simulink model "TTS2_EXT"  (R2025b)
settings: Solver=FixedStepAuto  StartTime=0.0  StopTime=inf  FixedStep=0.01  RelTol=1e-3
model workspace (MAT data in the model file):
  amp_f1 = -100
  amp_f10 = 0.5
  amp_f11 = -0.1
  amp_f12 = 1
  amp_f13 = 0.5
  amp_f14 = -20
  amp_f15 = 0.5
  amp_f16 = 0.5
  amp_f17 = 20
  amp_f18 = -30
  amp_f19 = 0.1
  amp_f2 = -20
  amp_f20 = -20
  amp_f21 = 20
  amp_f3 = -30
  amp_f4 = -30
  amp_f5 = -10
  amp_f51 = -10
  amp_f52 = -30
  amp_f53 = -30
  amp_f54 = 20
  amp_f55 = -100
  amp_f6 = -30
  amp_f7 = -30
  amp_f8 = -30
  amp_f9 = 1
  from_f1 = 570
  from_f10 = 5970
  from_f11 = 6570
  from_f12 = 7170
  from_f13 = 7770
  from_f14 = 8370
  from_f15 = 8970
  from_f16 = 9570
  from_f17 = 10170
  from_f18 = 10770
  from_f19 = 11370
  from_f2 = 1170
  from_f20 = 11970
  from_f21 = 12570
  from_f3 = 1770
  from_f4 = 2370
  from_f5 = 2970
  from_f51 = 13170
  from_f52 = 13770
  from_f53 = 14370
  from_f54 = 14970
  from_f55 = 15570
  from_f6 = 3570
  from_f7 = 4170
  from_f8 = 4770
  from_f9 = 5370
libraries: lab310_library x26, neural x15, simulink x4, opclib x3, fuzblock x1
(part 2 of 3)

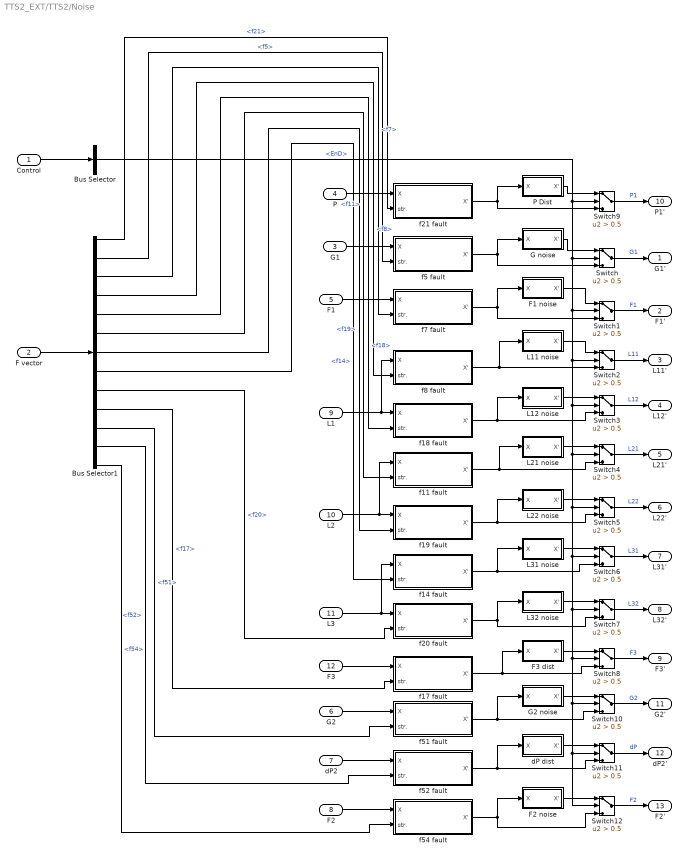
== system TTS2_EXT/TTS2/Noise ==
  Control : Inport
  F vector : Inport  Port=2
  G1 : Inport  Port=3
  P : Inport  Port=4
  F1 : Inport  Port=5
  G2 : Inport  Port=6
  dP2 : Inport  Port=7
  F2 : Inport  Port=8
  L1 : Inport  Port=9
  L2 : Inport  Port=10
  L3 : Inport  Port=11
  F3 : Inport  Port=12
  Bus Selector : BusSelector  OutputSignals=EnD
  Bus Selector1 : BusSelector  OutputSignals=f21,f5,f7,f8,f18,f11,f19,f14,f20,f17,f51,f52,f54
  F1 noise : Subsystem
  F2 noise : Subsystem
  F3 dist : Subsystem
  G noise : Subsystem
  G2 noise : Subsystem
  L11 noise : Subsystem
  L12 noise : Subsystem
  L21 noise : Subsystem
  L22 noise : Subsystem
  L31 noise : Subsystem
  L32 noise : Subsystem
  P Dist : Subsystem
  Switch{,1..12} (13 alike) : Switch  Criteria=u2 > Threshold  Threshold=0.5  SaturateOnIntegerOverflow=off  InputSameDT=off
  dP dist : Subsystem
  f11 fault : Subsystem
  f14 fault : Subsystem
  f17 fault : Subsystem
  f18 fault : Subsystem
  f19 fault : Subsystem
  f20 fault : Subsystem
  f21 fault : Subsystem
  f5 fault : Subsystem
  f51 fault : Subsystem
  f52 fault : Subsystem
  f54 fault : Subsystem
  f7 fault : Subsystem
  f8 fault : Subsystem
  G1' : Outport  VectorParamsAs1DForOutWhenUnconnected=off
  F1' : Outport  Port=2  VectorParamsAs1DForOutWhenUnconnected=off
  L11' : Outport  Port=3  VectorParamsAs1DForOutWhenUnconnected=off
  L12' : Outport  Port=4  VectorParamsAs1DForOutWhenUnconnected=off
  L21' : Outport  Port=5  VectorParamsAs1DForOutWhenUnconnected=off
  L22' : Outport  Port=6  VectorParamsAs1DForOutWhenUnconnected=off
  L31' : Outport  Port=7  VectorParamsAs1DForOutWhenUnconnected=off
  L32' : Outport  Port=8  VectorParamsAs1DForOutWhenUnconnected=off
  F3' : Outport  Port=9  VectorParamsAs1DForOutWhenUnconnected=off
  P1' : Outport  Port=10  VectorParamsAs1DForOutWhenUnconnected=off
  G2' : Outport  Port=11  VectorParamsAs1DForOutWhenUnconnected=off
  dP2' : Outport  Port=12  VectorParamsAs1DForOutWhenUnconnected=off
  F2' : Outport  Port=13  VectorParamsAs1DForOutWhenUnconnected=off
  wires:
  f21 fault/1(X') -> P Dist/1(X), Switch9/3
  P Dist/1(X') -> Switch9/1
  Switch9/1 -> P1'/1  "P1"
  P/1 -> f21 fault/1(X)
  Switch2/1 -> L11'/1  "L11"
  Switch8/1 -> F3'/1  "F3"
  Switch7/1 -> L32'/1  "L32"
  F1 noise/1(X') -> Switch1/1
  Switch3/1 -> L12'/1  "L12"
  Switch4/1 -> L21'/1  "L21"
  Switch6/1 -> L31'/1  "L31"
  L11 noise/1(X') -> Switch2/1
  G noise/1(X') -> Switch/1
  Switch5/1 -> L22'/1  "L22"
  f20 fault/1(X') -> Switch7/3, L32 noise/1(X)
  F3 dist/1(X') -> Switch8/1
  f11 fault/1(X') -> Switch4/3, L21 noise/1(X)
  L32 noise/1(X') -> Switch7/1
  L31 noise/1(X') -> Switch6/1
  f18 fault/1(X') -> Switch3/3, L12 noise/1(X)
  F1/1 -> f7 fault/1(X)
  L22 noise/1(X') -> Switch5/1
  L1/1 -> f18 fault/1(X), f8 fault/1(X)
  L2/1 -> f11 fault/1(X), f19 fault/1(X)
  Switch/1 -> G1'/1  "G1"
  f5 fault/1(X') -> Switch/3, G noise/1(X)
  L21 noise/1(X') -> Switch4/1
  f19 fault/1(X') -> Switch5/3, L22 noise/1(X)
  Bus Selector/1 -> Switch9/2, Switch8/2, Switch12/2, Switch11/2, Switch10/2, Switch7/2, Switch6/2, Switch5/2, Switch4/2, Switch3/2, Switch2/2, Switch1/2, Switch/2  "<EnD>"
  f17 fault/1(X') -> F3 dist/1(X), Switch8/3
  Switch1/1 -> F1'/1  "F1"
  L12 noise/1(X') -> Switch3/1
  f8 fault/1(X') -> Switch2/3, L11 noise/1(X)
  f14 fault/1(X') -> Switch6/3, L31 noise/1(X)
  f7 fault/1(X') -> Switch1/3, F1 noise/1(X)
  L3/1 -> f14 fault/1(X), f20 fault/1(X)
  G1/1 -> f5 fault/1(X)
  Control/1 -> Bus Selector/1
  F vector/1 -> Bus Selector1/1
  Bus Selector1/1 -> f21 fault/2(str.)  "<f21>"
  Bus Selector1/2 -> f5 fault/2(str.)  "<f5>"
  Bus Selector1/3 -> f7 fault/2(str.)  "<f7>"
  Bus Selector1/4 -> f8 fault/2(str.)  "<f8>"
  Bus Selector1/5 -> f18 fault/2(str.)  "<f18>"
  Bus Selector1/6 -> f11 fault/2(str.)  "<f11>"
  Bus Selector1/7 -> f19 fault/2(str.)  "<f19>"
  Bus Selector1/8 -> f14 fault/2(str.)  "<f14>"
  Bus Selector1/9 -> f20 fault/2(str.)  "<f20>"
  Bus Selector1/10 -> f17 fault/2(str.)  "<f17>"
  dP2/1 -> f52 fault/1(X)
  G2/1 -> f51 fault/1(X)
  Switch12/1 -> F2'/1  "F2"
  Switch11/1 -> dP2'/1  "dP"
  Switch10/1 -> G2'/1  "G2"
  f54 fault/1(X') -> F2 noise/1(X), Switch12/3
  f52 fault/1(X') -> Switch11/3, dP dist/1(X)
  f51 fault/1(X') -> Switch10/3, G2 noise/1(X)
  G2 noise/1(X') -> Switch10/1
  dP dist/1(X') -> Switch11/1
  F2 noise/1(X') -> Switch12/1
  Bus Selector1/11 -> f51 fault/2(str.)  "<f51>"
  Bus Selector1/12 -> f52 fault/2(str.)  "<f52>"
  Bus Selector1/13 -> f54 fault/2(str.)  "<f54>"
  F2/1 -> f54 fault/1(X)
  F3/1 -> f17 fault/1(X)

== system TTS2_EXT/TTS2/Pump+pipe+control valve ==
  CV1 : Inport
  F vec : Inport  Port=2
  CV2 : Inport  Port=3
  Add : Sum
  Bus Selector : BusSelector  OutputSignals=f1,f2,f4,f6,f53
  Patm[kPa] : Constant  Value=1.013  OutMin=[0.1013]  OutMax=[2.026]
  Pump control [%] : Constant  Value=pc  mask{pc=100.0}
      mask prompts: pc "Pump control"
  Pump+Pipe : Subsystem
  V1 : Subsystem
  V2 : Subsystem
  f1 fault : Subsystem
  f2 fault : Subsystem
  X1[%] : Outport  VectorParamsAs1DForOutWhenUnconnected=off
  F1[m3/s] : Outport  Port=2  VectorParamsAs1DForOutWhenUnconnected=off
  dP1[kPa] : Outport  Port=3  VectorParamsAs1DForOutWhenUnconnected=off
  P[kPa] : Outport  Port=4  VectorParamsAs1DForOutWhenUnconnected=off
  X2[%] : Outport  Port=5  VectorParamsAs1DForOutWhenUnconnected=off
  F2[m3/s] : Outport  Port=6  VectorParamsAs1DForOutWhenUnconnected=off
  dP2[kPa] : Outport  Port=7  VectorParamsAs1DForOutWhenUnconnected=off
  wires:
  Pump control [%]/1 -> f1 fault/1(X)
  f2 fault/1(Xf) -> Pump+Pipe/1(MP)
  f1 fault/1(Xf) -> f2 fault/1(X)
  Bus Selector/2 -> f2 fault/2(str.)  "<f2>"
  Bus Selector/1 -> f1 fault/2(str.)  "<f1>"
  F vec/1 -> Bus Selector/1
  Pump+Pipe/1(P[kPa]) -> P[kPa]/1, V2/2(P1[kPa]), V1/2(P1[kPa])
  CV1/1 -> V1/1(CV[%])
  Patm[kPa]/1 -> V2/3(P2[kPa]), V1/3(P2[kPa])
  Bus Selector/3 -> V1/4(f04)  "<f4>"
  Bus Selector/4 -> V1/5(f06)  "<f6>"
  V1/1(X[%]) -> X1[%]/1
  V1/3(dP[kPa]) -> dP1[kPa]/1
  V1/2(F[m3/s]) -> Add/2, F1[m3/s]/1
  CV2/1 -> V2/1(CV[%])
  V2/1(X[%]) -> X2[%]/1
  V2/2(F[m3/s]) -> Add/1, F2[m3/s]/1
  V2/3(dP[kPa]) -> dP2[kPa]/1
  Bus Selector/5 -> V2/4(f53)  "<f53>"
  Add/1 -> Pump+Pipe/2(F[m3/h])

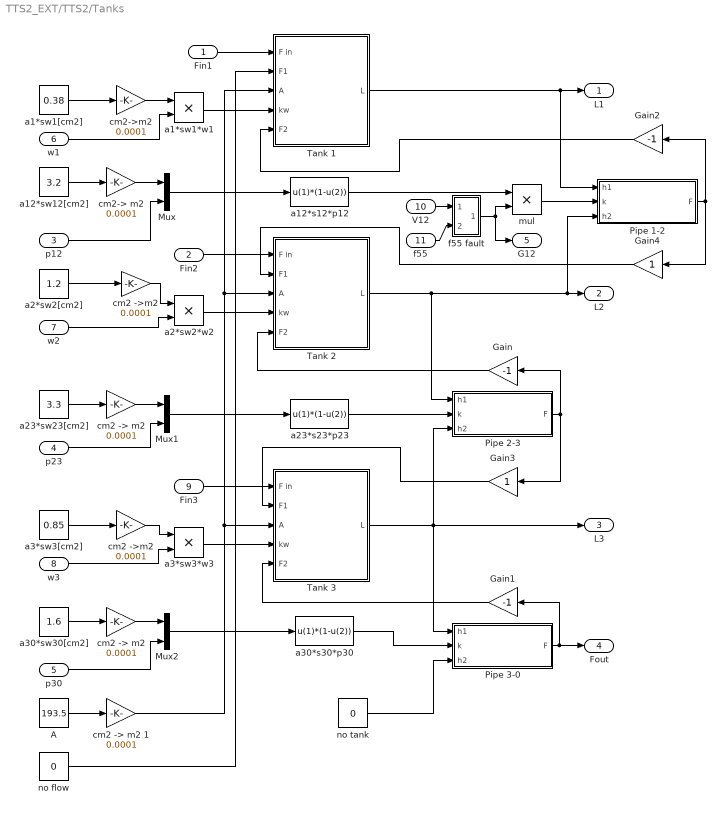
== system TTS2_EXT/TTS2/Tanks ==
  Fin1 : Inport
  Fin2 : Inport  Port=2
  p12 : Inport  Port=3
  p23 : Inport  Port=4
  p30 : Inport  Port=5
  w1 : Inport  Port=6
  w2 : Inport  Port=7
  w3 : Inport  Port=8
  Fin3 : Inport  Port=9
  V12 : Inport  Port=10
  f55 : Inport  Port=11
  A : Constant  Value=193.5
  Gain : Gain  Gain=-1
  Gain1 : Gain  Gain=-1
  Gain2 : Gain  Gain=-1
  Gain3 : Gain
  Gain4 : Gain
  Mux : Mux  Inputs=2
  Mux1 : Mux  Inputs=2
  Mux2 : Mux  Inputs=2
  Pipe 1-2 : Subsystem
  Pipe 2-3 : Subsystem
  Pipe 3-0 : Subsystem
  "Tank 1 " : Subsystem
  Tank 2 : Subsystem
  Tank 3 : Subsystem
  a1*sw1*w1 : Product
  a1*sw1[cm2] : Constant  Value=0.38
  a12*s12*p12 : Fcn  Expr=u(1)*(1-u(2))
  a12*sw12[cm2] : Constant  Value=3.2
  a2*sw2*w2 : Product
  a2*sw2[cm2] : Constant  Value=1.2
  a23*s23*p23 : Fcn  Expr=u(1)*(1-u(2))
  a23*sw23[cm2] : Constant  Value=3.3
  a3*sw3*w3 : Product
  a3*sw3[cm2] : Constant  Value=0.85
  a30*s30*p30 : Fcn  Expr=u(1)*(1-u(2))
  a30*sw30[cm2] : Constant  Value=1.6
  "cm2 -> m2" : Gain  Gain=0.0001
  "cm2 -> m2 " : Gain  Gain=0.0001
  "cm2 -> m2 1" : Gain  Gain=0.0001
  cm2 ->m2 : Gain  Gain=0.0001
  "cm2 ->m2 " : Gain  Gain=0.0001
  cm2-> m2 : Gain  Gain=0.0001
  cm2->m2 : Gain  Gain=0.0001
  f55 fault : Subsystem
  mul : Product
  no flow : Constant  Value=0
  no tank : Constant  Value=0
  L1 : Outport  VectorParamsAs1DForOutWhenUnconnected=off
  L2 : Outport  Port=2  VectorParamsAs1DForOutWhenUnconnected=off
  L3 : Outport  Port=3  VectorParamsAs1DForOutWhenUnconnected=off
  Fout : Outport  Port=4  VectorParamsAs1DForOutWhenUnconnected=off
  G12 : Outport  Port=5  VectorParamsAs1DForOutWhenUnconnected=off
  wires:
  Fin1/1 -> "Tank 1 "/1(F in)
  a1*sw1[cm2]/1 -> cm2->m2/1
  cm2->m2/1 -> a1*sw1*w1/1
  a1*sw1*w1/1 -> "Tank 1 "/4(kw)
  w1/1 -> a1*sw1*w1/2
  a12*sw12[cm2]/1 -> cm2-> m2/1
  cm2-> m2/1 -> Mux/1
  p12/1 -> Mux/2
  Mux/1 -> a12*s12*p12/1
  a2*sw2[cm2]/1 -> cm2 ->m2/1
  cm2 ->m2/1 -> a2*sw2*w2/1
  a23*sw23[cm2]/1 -> "cm2 -> m2"/1
  "cm2 -> m2"/1 -> Mux1/1
  Mux1/1 -> a23*s23*p23/1
  w2/1 -> a2*sw2*w2/2
  p23/1 -> Mux1/2
  a2*sw2*w2/1 -> Tank 2/4(kw)
  a3*sw3[cm2]/1 -> "cm2 ->m2 "/1
  "cm2 ->m2 "/1 -> a3*sw3*w3/1
  a30*sw30[cm2]/1 -> "cm2 -> m2 "/1
  "cm2 -> m2 "/1 -> Mux2/1
  w3/1 -> a3*sw3*w3/2
  p30/1 -> Mux2/2
  Mux2/1 -> a30*s30*p30/1
  a3*sw3*w3/1 -> Tank 3/4(kw)
  A/1 -> "cm2 -> m2 1"/1
  no flow/1 -> "Tank 1 "/2(F1)
  "cm2 -> m2 1"/1 -> Tank 3/3(A), Tank 2/3(A), "Tank 1 "/3(A)
  "Tank 1 "/1(L) -> Pipe 1-2/1(h1), L1/1
  a12*s12*p12/1 -> mul/1
  Tank 2/1(L) -> Pipe 1-2/3(h2), L2/1, Pipe 2-3/1(h1)
  a23*s23*p23/1 -> Pipe 2-3/2(k)
  Tank 3/1(L) -> Pipe 2-3/3(h2), Pipe 3-0/1(h1), L3/1
  a30*s30*p30/1 -> Pipe 3-0/2(k)
  no tank/1 -> Pipe 3-0/3(h2)
  Pipe 3-0/1(F) -> Fout/1, Gain1/1
  Pipe 2-3/1(F) -> Gain3/1, Gain/1
  Pipe 1-2/1(F) -> Gain2/1, Gain4/1
  Gain2/1 -> "Tank 1 "/5(F2)
  Gain/1 -> Tank 2/5(F2)
  Fin3/1 -> Tank 3/1(F in)
  Gain1/1 -> Tank 3/5(F2)
  Gain3/1 -> Tank 3/2(F1)
  Gain4/1 -> Tank 2/2(F1)
  Fin2/1 -> Tank 2/1(F in)
  mul/1 -> Pipe 1-2/2(k)
  V12/1 -> f55 fault/1(X)
  f55/1 -> f55 fault/2(str.)
  f55 fault/1(X') -> G12/1, mul/2

== system TTS2_EXT/TTS2/f3 fault ==
  X : Inport
  str. : Inport  Port=2
  Add : Sum
  Fcn : Fcn  Expr=u(1)*((u(2)/100)+1)
  Manual Switch : ManualSwitch  CurrentSetting=0
  Mux : Mux  Inputs=2
  X' : Outport  VectorParamsAs1DForOutWhenUnconnected=off
  wires:
  Mux/1 -> Fcn/1
  X/1 -> Add/1, Mux/1
  str./1 -> Add/2, Mux/2
  Manual Switch/1 -> X'/1
  Add/1 -> Manual Switch/1
  Fcn/1 -> Manual Switch/2

== system TTS2_EXT/Monitoring & Analysis/r4/Function Fitting Neural Network ==
  Input : Inport  PortDimensions=1
      mask Display: e = 0.06;c1 = [120 230 180]/255;c2 = ([120 230 180]+0)/(256+128);c3 = ([120 230 180]+128)/(256+128);patch([0 1 1 0],[0 0 1 1],c1);patch([0 1 1 1-e 1-e 0+e],[0 0 1 1-e 0+e 0+e],c2);patch([0 0 1 1-e 0+e 0+e],[0 1 1 1-e 1-e 0+e],c3);plot([0 1 1 0 0],[0 0 1 1 0]);
  Layer 1 : Subsystem
      mask Display: e = 0.06;c1 = [120 150 230]/255;c2 = ([120 150 230]+0)/383;c3 = ([120 150 230]+128)/383;patch([0 1 1 0],[0 0 1 1],c1);patch([0 1 1 1-e 1-e 0+e],[0 0 1 1-e 0+e 0+e],c2);patch([0 0 1 1-e 0+e 0+e],[0 1 1 1-e 1-e 0+e],c3);plot([0 1 1 0 0],[0 0 1 1 0]);
  Layer 2 : Subsystem
      mask Display: e = 0.06;c1 = [120 150 230]/255;c2 = ([120 150 230]+0)/383;c3 = ([120 150 230]+128)/383;patch([0 1 1 0],[0 0 1 1],c1);patch([0 1 1 1-e 1-e 0+e],[0 0 1 1-e 0+e 0+e],c2);patch([0 0 1 1-e 0+e 0+e],[0 1 1 1-e 1-e 0+e],c3);plot([0 1 1 0 0],[0 0 1 1 0]);
  Process Input 1 : Subsystem
      mask Display: e = 0.06;c1 = [120 150 230]/255;c2 = ([120 150 230]+0)/383;c3 = ([120 150 230]+128)/383;patch([0 1 1 0],[0 0 1 1],c1);patch([0 1 1 1-e 1-e 0+e],[0 0 1 1-e 0+e 0+e],c2);patch([0 0 1 1-e 0+e 0+e],[0 1 1 1-e 1-e 0+e],c3);plot([0 1 1 0 0],[0 0 1 1 0]);
  Process Output 1 : Subsystem
      mask Display: e = 0.06;c1 = [120 150 230]/255;c2 = ([120 150 230]+0)/383;c3 = ([120 150 230]+128)/383;patch([0 1 1 0],[0 0 1 1],c1);patch([0 1 1 1-e 1-e 0+e],[0 0 1 1-e 0+e 0+e],c2);patch([0 0 1 1-e 0+e 0+e],[0 1 1 1-e 1-e 0+e],c3);plot([0 1 1 0 0],[0 0 1 1 0]);
  Output : Outport  InitialOutput=0
      mask Display: e = 0.06;c1 = [120 230 180]/255;c2 = ([120 230 180]+0)/(256+128);c3 = ([120 230 180]+128)/(256+128);patch([0 1 1 0],[0 0 1 1],c1);patch([0 1 1 1-e 1-e 0+e],[0 0 1 1-e 0+e 0+e],c2);patch([0 0 1 1-e 0+e 0+e],[0 1 1 1-e 1-e 0+e],c3);plot([0 1 1 0 0],[0 0 1 1 0]);
  wires:
  Input/1 -> Process Input 1/1(x)
  Process Output 1/1(y) -> Output/1
  Process Input 1/1(p) -> Layer 1/1("p{1}")
  Layer 1/1("a{1}") -> [feedback1]
  [feedback1] -> Layer 2/1("a{1} ")
  Layer 2/1("a{2}") -> Process Output 1/1(a)

== system TTS2_EXT/Subsystem1/PID/Antiwindup ==
  CV : Inport
  Logical Operator : Logic  Operator=NOR  AllPortsSameDT=off  OutDataTypeStr=boolean
  Relational Operator : RelationalOperator  Operator=<=  OutDataTypeStr=boolean  RndMeth=Simplest  InputSameDT=off
  Relational Operator1 : RelationalOperator  OutDataTypeStr=boolean  RndMeth=Simplest  InputSameDT=off
  norm CV max : Constant
  norm CVmin : Constant  Value=0
  enable : Outport  VectorParamsAs1DForOutWhenUnconnected=off
  wires:
  norm CVmin/1 -> Relational Operator/2
  norm CV max/1 -> Relational Operator1/2
  CV/1 -> Relational Operator1/1, Relational Operator/1
  Relational Operator/1 -> Logical Operator/1
  Relational Operator1/1 -> Logical Operator/2
  Logical Operator/1 -> enable/1

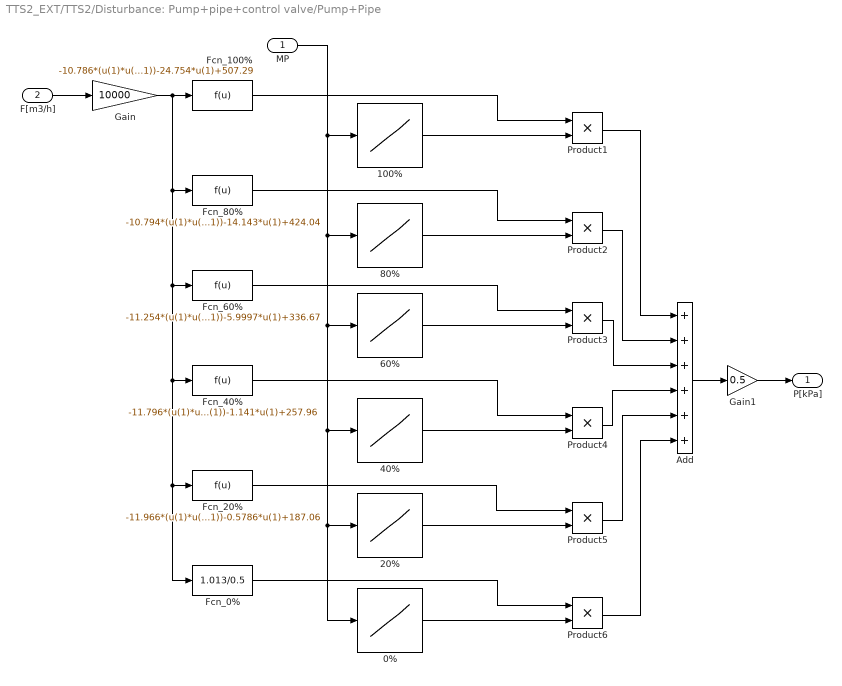
== system TTS2_EXT/TTS2/Disturbance: Pump+pipe+control valve/Pump+Pipe ==
  MP : Inport
  F[m3/h] : Inport  Port=2
  "0% " : Lookup_n-D  NumberOfTableDimensions=1  BreakpointsForDimension1=[0 20 100]  Table=[1 0 0]  InternalRulePriority=Speed  RndMeth=Simplest
  100% : Lookup_n-D  NumberOfTableDimensions=1  BreakpointsForDimension1=[0 80 100]  Table=[0 0 1]  InternalRulePriority=Speed  RndMeth=Simplest
  20% : Lookup_n-D  NumberOfTableDimensions=1  BreakpointsForDimension1=[0 20 40 100]  Table=[0 1 0 0]  InternalRulePriority=Speed  RndMeth=Simplest
  40% : Lookup_n-D  NumberOfTableDimensions=1  BreakpointsForDimension1=[0 20 40 60 100]  Table=[0 0 1 0 0]  InternalRulePriority=Speed  RndMeth=Simplest
  60% : Lookup_n-D  NumberOfTableDimensions=1  BreakpointsForDimension1=[0 40 60 80 100]  Table=[0 0 1 0 0]  InternalRulePriority=Speed  RndMeth=Simplest
  80% : Lookup_n-D  NumberOfTableDimensions=1  BreakpointsForDimension1=[0 60 80 100]  Table=[0 0 1 0]  InternalRulePriority=Speed  RndMeth=Simplest
  Add : Sum  Inputs=6
  Fcn_0% : Fcn  Expr=1.013/0.5
  Fcn_100% : Fcn  Expr=-10.786*(u(1)*u(1))-24.754*u(1)+507.29
  Fcn_20% : Fcn  Expr=-11.966*(u(1)*u(1))-0.5786*u(1)+187.06
  Fcn_40% : Fcn  Expr=-11.796*(u(1)*u(1))-1.141*u(1)+257.96
  Fcn_60% : Fcn  Expr=-11.254*(u(1)*u(1))-5.9997*u(1)+336.67
  Fcn_80% : Fcn  Expr=-10.794*(u(1)*u(1))-14.143*u(1)+424.04
  Gain : Gain  Gain=10000
  Gain1 : Gain  Gain=0.5
  Product{1..6} (6 alike) : Product
  P[kPa] : Outport  VectorParamsAs1DForOutWhenUnconnected=off
  wires:
  F[m3/h]/1 -> Gain/1
  MP/1 -> 80%/1, 40%/1, 20%/1, "0% "/1, 60%/1, 100%/1
  "0% "/1 -> Product6/2
  20%/1 -> Product5/2
  40%/1 -> Product4/2
  60%/1 -> Product3/2
  80%/1 -> Product2/2
  100%/1 -> Product1/2
  Gain/1 -> Fcn_20%/1, Fcn_0%/1, Fcn_40%/1, Fcn_60%/1, Fcn_80%/1, Fcn_100%/1
  Fcn_0%/1 -> Product6/1
  Fcn_20%/1 -> Product5/1
  Fcn_40%/1 -> Product4/1
  Fcn_60%/1 -> Product3/1
  Fcn_80%/1 -> Product2/1
  Fcn_100%/1 -> Product1/1
  Product1/1 -> Add/1
  Product2/1 -> Add/2
  Product3/1 -> Add/3
  Product4/1 -> Add/4
  Product5/1 -> Add/5
  Product6/1 -> Add/6
  Add/1 -> Gain1/1
  Gain1/1 -> P[kPa]/1

== system TTS2_EXT/TTS2/Disturbance: Pump+pipe+control valve/VB ==
  CV[%] : Inport
  P1[kPa] : Inport  Port=2
  P2[kPa] : Inport  Port=3
  Positioner : Subsystem
  Valve : Subsystem
  F[m3/h] : Outport  VectorParamsAs1DForOutWhenUnconnected=off
  wires:
  Valve/1(F[m3/h]) -> F[m3/h]/1
  P1[kPa]/1 -> Valve/2(P1[kPa])
  P2[kPa]/1 -> Valve/3(P2[kPa])
  CV[%]/1 -> Positioner/1(CV[0-100])
  Positioner/1(X[0-1]) -> Valve/1(G[0-1])

== system TTS2_EXT/TTS2/Noise/F1 noise ==
  X : Inport
  Random Number : RandomNumber  Variance=0.006889  Seed=3341  SampleTime=1
  Sum : Sum  Inputs=|++
  X' : Outport  VectorParamsAs1DForOutWhenUnconnected=off
  wires:
  Random Number/1 -> Sum/2
  X/1 -> Sum/1
  Sum/1 -> X'/1

== system TTS2_EXT/TTS2/Noise/F2 noise ==
  X : Inport
  Random Number : RandomNumber  Variance=0.0225  Seed=765756  SampleTime=1
  Sum : Sum  Inputs=|++
  X' : Outport  VectorParamsAs1DForOutWhenUnconnected=off
  wires:
  Random Number/1 -> Sum/2
  X/1 -> Sum/1
  Sum/1 -> X'/1

== system TTS2_EXT/TTS2/Noise/F3 dist ==
  X : Inport
  Random Number : RandomNumber  Variance=0.0225  Seed=756756  SampleTime=1
  Sum : Sum  Inputs=|++
  X' : Outport  VectorParamsAs1DForOutWhenUnconnected=off
  wires:
  Random Number/1 -> Sum/2
  X/1 -> Sum/1
  Sum/1 -> X'/1

== system TTS2_EXT/TTS2/Noise/G noise ==
  X : Inport
  Random Number : RandomNumber  Variance=0.006889  Seed=2312  SampleTime=1
  Sum : Sum  Inputs=|++
  X' : Outport  VectorParamsAs1DForOutWhenUnconnected=off
  wires:
  Random Number/1 -> Sum/2
  X/1 -> Sum/1
  Sum/1 -> X'/1

== system TTS2_EXT/TTS2/Noise/G2 noise ==
  X : Inport
  Random Number : RandomNumber  Variance=0.0225  Seed=75675675  SampleTime=1
  Sum : Sum  Inputs=|++
  X' : Outport  VectorParamsAs1DForOutWhenUnconnected=off
  wires:
  Random Number/1 -> Sum/2
  X/1 -> Sum/1
  Sum/1 -> X'/1

== system TTS2_EXT/TTS2/Noise/L11 noise ==
  X : Inport
  Random Number : RandomNumber  Variance=0.000002777  Seed=4324  SampleTime=1
  Sum : Sum  Inputs=|++
  X' : Outport  VectorParamsAs1DForOutWhenUnconnected=off
  wires:
  Random Number/1 -> Sum/2
  X/1 -> Sum/1
  Sum/1 -> X'/1

== system TTS2_EXT/TTS2/Noise/L12 noise ==
  X : Inport
  Random Number : RandomNumber  Variance=0.00000053777  Seed=432423  SampleTime=1
  Sum : Sum  Inputs=|++
  X' : Outport  VectorParamsAs1DForOutWhenUnconnected=off
  wires:
  Random Number/1 -> Sum/2
  X/1 -> Sum/1
  Sum/1 -> X'/1

== system TTS2_EXT/TTS2/Noise/L21 noise ==
  X : Inport
  Random Number : RandomNumber  Variance=0.000000111111111  Seed=43243423  SampleTime=1
  Sum : Sum  Inputs=|++
  X' : Outport  VectorParamsAs1DForOutWhenUnconnected=off
  wires:
  Random Number/1 -> Sum/2
  X/1 -> Sum/1
  Sum/1 -> X'/1

== system TTS2_EXT/TTS2/Noise/L22 noise ==
  X : Inport
  Random Number : RandomNumber  Variance=0.0000001111111111  Seed=32423  SampleTime=1
  Sum : Sum  Inputs=|++
  X' : Outport  VectorParamsAs1DForOutWhenUnconnected=off
  wires:
  Random Number/1 -> Sum/2
  X/1 -> Sum/1
  Sum/1 -> X'/1

== system TTS2_EXT/TTS2/Noise/L31 noise ==
  X : Inport
  Random Number : RandomNumber  Variance=0.0000017777  Seed=432454  SampleTime=1
  Sum : Sum  Inputs=|++
  X' : Outport  VectorParamsAs1DForOutWhenUnconnected=off
  wires:
  Random Number/1 -> Sum/2
  X/1 -> Sum/1
  Sum/1 -> X'/1

== system TTS2_EXT/TTS2/Noise/L32 noise ==
  X : Inport
  Random Number : RandomNumber  Variance=0.0000006944  Seed=4563565  SampleTime=1
  Sum : Sum  Inputs=|++
  X' : Outport  VectorParamsAs1DForOutWhenUnconnected=off
  wires:
  Random Number/1 -> Sum/2
  X/1 -> Sum/1
  Sum/1 -> X'/1

== system TTS2_EXT/TTS2/Noise/P Dist ==
  X : Inport
  Random Number : RandomNumber  Variance=0.09  Seed=32321  SampleTime=1
  Sum : Sum  Inputs=|++
  X' : Outport  VectorParamsAs1DForOutWhenUnconnected=off
  wires:
  Random Number/1 -> Sum/2
  X/1 -> Sum/1
  Sum/1 -> X'/1

== system TTS2_EXT/TTS2/Noise/dP dist ==
  X : Inport
  Random Number : RandomNumber  Variance=0.09  Seed=756756756  SampleTime=1
  Sum : Sum  Inputs=|++
  X' : Outport  VectorParamsAs1DForOutWhenUnconnected=off
  wires:
  Random Number/1 -> Sum/2
  X/1 -> Sum/1
  Sum/1 -> X'/1

== system TTS2_EXT/TTS2/Noise/f11 fault ==
  X : Inport
  str. : Inport  Port=2
  Add : Sum
  Fcn : Fcn  Expr=u(1)*((u(2)/100)+1)
  Manual Switch : ManualSwitch
  Mux : Mux  Inputs=2
  X' : Outport  VectorParamsAs1DForOutWhenUnconnected=off
  wires:
  Mux/1 -> Fcn/1
  X/1 -> Add/1, Mux/1
  str./1 -> Add/2, Mux/2
  Add/1 -> Manual Switch/1
  Fcn/1 -> Manual Switch/2
  Manual Switch/1 -> X'/1

== system TTS2_EXT/TTS2/Noise/f14 fault ==
  X : Inport
  str. : Inport  Port=2
  Add : Sum
  Fcn : Fcn  Expr=u(1)*((u(2)/100)+1)
  Manual Switch : ManualSwitch  CurrentSetting=0
  Mux : Mux  Inputs=2
  X' : Outport  VectorParamsAs1DForOutWhenUnconnected=off
  wires:
  Mux/1 -> Fcn/1
  X/1 -> Add/1, Mux/1
  str./1 -> Add/2, Mux/2
  Add/1 -> Manual Switch/1
  Fcn/1 -> Manual Switch/2
  Manual Switch/1 -> X'/1

== system TTS2_EXT/TTS2/Noise/f17 fault ==
  X : Inport
  str. : Inport  Port=2
  Add : Sum
  Fcn : Fcn  Expr=u(1)*((u(2)/100)+1)
  Manual Switch : ManualSwitch  CurrentSetting=0
  Mux : Mux  Inputs=2
  X' : Outport  VectorParamsAs1DForOutWhenUnconnected=off
  wires:
  Mux/1 -> Fcn/1
  X/1 -> Add/1, Mux/1
  str./1 -> Add/2, Mux/2
  Add/1 -> Manual Switch/1
  Fcn/1 -> Manual Switch/2
  Manual Switch/1 -> X'/1

== system TTS2_EXT/TTS2/Noise/f18 fault ==
  X : Inport
  str. : Inport  Port=2
  Add : Sum
  Fcn : Fcn  Expr=u(1)*((u(2)/100)+1)
  Manual Switch : ManualSwitch  CurrentSetting=0
  Mux : Mux  Inputs=2
  X' : Outport  VectorParamsAs1DForOutWhenUnconnected=off
  wires:
  Mux/1 -> Fcn/1
  X/1 -> Add/1, Mux/1
  str./1 -> Add/2, Mux/2
  Fcn/1 -> Manual Switch/2
  Manual Switch/1 -> X'/1
  Add/1 -> Manual Switch/1

== system TTS2_EXT/TTS2/Noise/f19 fault ==
  X : Inport
  str. : Inport  Port=2
  Add : Sum
  Fcn : Fcn  Expr=u(1)*((u(2)/100)+1)
  Manual Switch : ManualSwitch
  Mux : Mux  Inputs=2
  X' : Outport  VectorParamsAs1DForOutWhenUnconnected=off
  wires:
  Mux/1 -> Fcn/1
  X/1 -> Add/1, Mux/1
  str./1 -> Add/2, Mux/2
  Add/1 -> Manual Switch/1
  Fcn/1 -> Manual Switch/2
  Manual Switch/1 -> X'/1

== system TTS2_EXT/TTS2/Noise/f20 fault ==
  X : Inport
  str. : Inport  Port=2
  Add : Sum
  Fcn : Fcn  Expr=u(1)*((u(2)/100)+1)
  Manual Switch : ManualSwitch  CurrentSetting=0
  Mux : Mux  Inputs=2
  X' : Outport  VectorParamsAs1DForOutWhenUnconnected=off
  wires:
  Mux/1 -> Fcn/1
  X/1 -> Add/1, Mux/1
  str./1 -> Add/2, Mux/2
  Add/1 -> Manual Switch/1
  Fcn/1 -> Manual Switch/2
  Manual Switch/1 -> X'/1

== system TTS2_EXT/TTS2/Noise/f21 fault ==
  X : Inport
  str. : Inport  Port=2
  Add : Sum
  Fcn : Fcn  Expr=u(1)*((u(2)/100)+1)
  Manual Switch : ManualSwitch  CurrentSetting=0
  Mux : Mux  Inputs=2
  X' : Outport  VectorParamsAs1DForOutWhenUnconnected=off
  wires:
  Mux/1 -> Fcn/1
  X/1 -> Add/1, Mux/1
  str./1 -> Add/2, Mux/2
  Add/1 -> Manual Switch/1
  Fcn/1 -> Manual Switch/2
  Manual Switch/1 -> X'/1

== system TTS2_EXT/TTS2/Noise/f5 fault ==
  X : Inport
  str. : Inport  Port=2
  Add : Sum
  Fcn : Fcn  Expr=u(1)*((u(2)/100)+1)
  Manual Switch : ManualSwitch
  Mux : Mux  Inputs=2
  X' : Outport  VectorParamsAs1DForOutWhenUnconnected=off
  wires:
  Mux/1 -> Fcn/1
  X/1 -> Add/1, Mux/1
  str./1 -> Add/2, Mux/2
  Add/1 -> Manual Switch/1
  Fcn/1 -> Manual Switch/2
  Manual Switch/1 -> X'/1

== system TTS2_EXT/TTS2/Noise/f51 fault ==
  X : Inport
  str. : Inport  Port=2
  Add : Sum
  Fcn : Fcn  Expr=u(1)*((u(2)/100)+1)
  Manual Switch : ManualSwitch
  Mux : Mux  Inputs=2
  X' : Outport  VectorParamsAs1DForOutWhenUnconnected=off
  wires:
  Mux/1 -> Fcn/1
  X/1 -> Add/1, Mux/1
  str./1 -> Add/2, Mux/2
  Add/1 -> Manual Switch/1
  Fcn/1 -> Manual Switch/2
  Manual Switch/1 -> X'/1

== system TTS2_EXT/TTS2/Noise/f52 fault ==
  X : Inport
  str. : Inport  Port=2
  Add : Sum
  Fcn : Fcn  Expr=u(1)*((u(2)/100)+1)
  Manual Switch : ManualSwitch  CurrentSetting=0
  Mux : Mux  Inputs=2
  X' : Outport  VectorParamsAs1DForOutWhenUnconnected=off
  wires:
  Mux/1 -> Fcn/1
  X/1 -> Add/1, Mux/1
  str./1 -> Add/2, Mux/2
  Add/1 -> Manual Switch/1
  Fcn/1 -> Manual Switch/2
  Manual Switch/1 -> X'/1

== system TTS2_EXT/TTS2/Noise/f54 fault ==
  X : Inport
  str. : Inport  Port=2
  Add : Sum
  Fcn : Fcn  Expr=u(1)*((u(2)/100)+1)
  Manual Switch : ManualSwitch  CurrentSetting=0
  Mux : Mux  Inputs=2
  X' : Outport  VectorParamsAs1DForOutWhenUnconnected=off
  wires:
  Mux/1 -> Fcn/1
  X/1 -> Add/1, Mux/1
  str./1 -> Add/2, Mux/2
  Add/1 -> Manual Switch/1
  Fcn/1 -> Manual Switch/2
  Manual Switch/1 -> X'/1

== system TTS2_EXT/TTS2/Noise/f7 fault ==
  X : Inport
  str. : Inport  Port=2
  Add : Sum
  Fcn : Fcn  Expr=u(1)*((u(2)/100)+1)
  Manual Switch : ManualSwitch  CurrentSetting=0
  Mux : Mux  Inputs=2
  X' : Outport  VectorParamsAs1DForOutWhenUnconnected=off
  wires:
  Mux/1 -> Fcn/1
  X/1 -> Add/1, Mux/1
  str./1 -> Add/2, Mux/2
  Add/1 -> Manual Switch/1
  Fcn/1 -> Manual Switch/2
  Manual Switch/1 -> X'/1

== system TTS2_EXT/TTS2/Noise/f8 fault ==
  X : Inport
  str. : Inport  Port=2
  Add : Sum
  Fcn : Fcn  Expr=u(1)*((u(2)/100)+1)
  Manual Switch : ManualSwitch  CurrentSetting=0
  Mux : Mux  Inputs=2
  X' : Outport  VectorParamsAs1DForOutWhenUnconnected=off
  wires:
  Mux/1 -> Fcn/1
  X/1 -> Add/1, Mux/1
  str./1 -> Add/2, Mux/2
  Add/1 -> Manual Switch/1
  Fcn/1 -> Manual Switch/2
  Manual Switch/1 -> X'/1

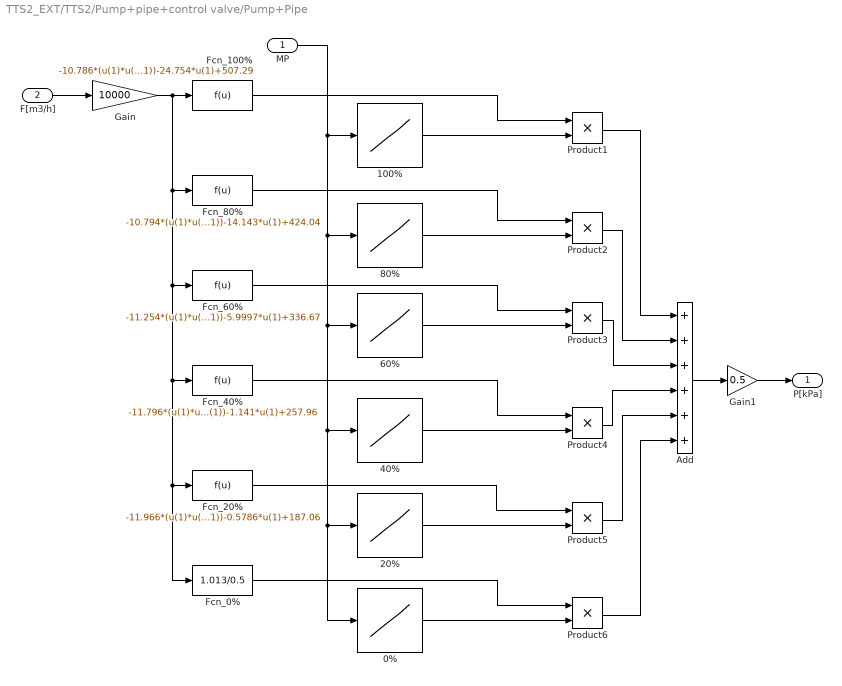
== system TTS2_EXT/TTS2/Pump+pipe+control valve/Pump+Pipe ==
  MP : Inport
  F[m3/h] : Inport  Port=2
  "0% " : Lookup_n-D  NumberOfTableDimensions=1  BreakpointsForDimension1=[0 20 100]  Table=[1 0 0]  InternalRulePriority=Speed  RndMeth=Simplest
  100% : Lookup_n-D  NumberOfTableDimensions=1  BreakpointsForDimension1=[0 80 100]  Table=[0 0 1]  InternalRulePriority=Speed  RndMeth=Simplest
  20% : Lookup_n-D  NumberOfTableDimensions=1  BreakpointsForDimension1=[0 20 40 100]  Table=[0 1 0 0]  InternalRulePriority=Speed  RndMeth=Simplest
  40% : Lookup_n-D  NumberOfTableDimensions=1  BreakpointsForDimension1=[0 20 40 60 100]  Table=[0 0 1 0 0]  InternalRulePriority=Speed  RndMeth=Simplest
  60% : Lookup_n-D  NumberOfTableDimensions=1  BreakpointsForDimension1=[0 40 60 80 100]  Table=[0 0 1 0 0]  InternalRulePriority=Speed  RndMeth=Simplest
  80% : Lookup_n-D  NumberOfTableDimensions=1  BreakpointsForDimension1=[0 60 80 100]  Table=[0 0 1 0]  InternalRulePriority=Speed  RndMeth=Simplest
  Add : Sum  Inputs=6
  Fcn_0% : Fcn  Expr=1.013/0.5
  Fcn_100% : Fcn  Expr=-10.786*(u(1)*u(1))-24.754*u(1)+507.29
  Fcn_20% : Fcn  Expr=-11.966*(u(1)*u(1))-0.5786*u(1)+187.06
  Fcn_40% : Fcn  Expr=-11.796*(u(1)*u(1))-1.141*u(1)+257.96
  Fcn_60% : Fcn  Expr=-11.254*(u(1)*u(1))-5.9997*u(1)+336.67
  Fcn_80% : Fcn  Expr=-10.794*(u(1)*u(1))-14.143*u(1)+424.04
  Gain : Gain  Gain=10000
  Gain1 : Gain  Gain=0.5
  Product{1..6} (6 alike) : Product
  P[kPa] : Outport  VectorParamsAs1DForOutWhenUnconnected=off
  wires:
  F[m3/h]/1 -> Gain/1
  MP/1 -> 80%/1, 40%/1, 20%/1, "0% "/1, 60%/1, 100%/1
  "0% "/1 -> Product6/2
  20%/1 -> Product5/2
  40%/1 -> Product4/2
  60%/1 -> Product3/2
  80%/1 -> Product2/2
  100%/1 -> Product1/2
  Gain/1 -> Fcn_20%/1, Fcn_0%/1, Fcn_40%/1, Fcn_60%/1, Fcn_80%/1, Fcn_100%/1
  Fcn_0%/1 -> Product6/1
  Fcn_20%/1 -> Product5/1
  Fcn_40%/1 -> Product4/1
  Fcn_60%/1 -> Product3/1
  Fcn_80%/1 -> Product2/1
  Fcn_100%/1 -> Product1/1
  Product1/1 -> Add/1
  Product2/1 -> Add/2
  Product3/1 -> Add/3
  Product4/1 -> Add/4
  Product5/1 -> Add/5
  Product6/1 -> Add/6
  Add/1 -> Gain1/1
  Gain1/1 -> P[kPa]/1

== system TTS2_EXT/TTS2/Pump+pipe+control valve/V1 ==
  CV[%] : Inport
  P1[kPa] : Inport  Port=2
  P2[kPa] : Inport  Port=3
  f04 : Inport  Port=4
  f06 : Inport  Port=5
  Gain2 : Gain  Gain=100
  Positioner : Subsystem
  Saturation : Saturate  UpperLimit=1  LowerLimit=0
  Valve : Subsystem
  f4 fault : Subsystem
  f6 fault : Subsystem
  X[%] : Outport  VectorParamsAs1DForOutWhenUnconnected=off
  F[m3/s] : Outport  Port=2  VectorParamsAs1DForOutWhenUnconnected=off
  dP[kPa] : Outport  Port=3  VectorParamsAs1DForOutWhenUnconnected=off
  wires:
  Valve/1(dP[kPa]) -> dP[kPa]/1
  Valve/2(F[m3/s]) -> F[m3/s]/1
  P1[kPa]/1 -> Valve/2(P1[kPa])
  P2[kPa]/1 -> Valve/3(P2[kPa])
  f06/1 -> f6 fault/2(str.)
  f6 fault/1(Xf) -> Saturation/1
  f4 fault/1(Xf) -> Positioner/1(CV[0-100])
  f04/1 -> f4 fault/2(str.)
  Positioner/1(X[0-1]) -> f6 fault/1(X), Gain2/1
  CV[%]/1 -> f4 fault/1(X)
  Gain2/1 -> X[%]/1
  Saturation/1 -> Valve/1(G[0-1])

== system TTS2_EXT/TTS2/Pump+pipe+control valve/V2 ==
  CV[%] : Inport
  P1[kPa] : Inport  Port=2
  P2[kPa] : Inport  Port=3
  f53 : Inport  Port=4
  Gain2 : Gain  Gain=100
  Positioner : Subsystem
  Saturation : Saturate  UpperLimit=1  LowerLimit=0
  Valve : Subsystem
  f53 fault : Subsystem
  X[%] : Outport  VectorParamsAs1DForOutWhenUnconnected=off
  F[m3/s] : Outport  Port=2  VectorParamsAs1DForOutWhenUnconnected=off
  dP[kPa] : Outport  Port=3  VectorParamsAs1DForOutWhenUnconnected=off
  wires:
  Valve/1(dP[kPa]) -> dP[kPa]/1
  Valve/2(F[m3/s]) -> F[m3/s]/1
  P1[kPa]/1 -> Valve/2(P1[kPa])
  P2[kPa]/1 -> Valve/3(P2[kPa])
  f53/1 -> f53 fault/2(str.)
  f53 fault/1(Xf) -> Saturation/1
  CV[%]/1 -> Positioner/1(CV[0-100])
  Positioner/1(X[0-1]) -> f53 fault/1(X), Gain2/1
  Gain2/1 -> X[%]/1
  Saturation/1 -> Valve/1(G[0-1])

== system TTS2_EXT/TTS2/Pump+pipe+control valve/f1 fault ==
  X : Inport
  str. : Inport  Port=2
  Add : Sum
  Fcn1 : Fcn  Expr=u(1)*((u(2)/100)+1)
  Manual Switch : ManualSwitch  CurrentSetting=0
  Mux1 : Mux  Inputs=2
  Xf : Outport  VectorParamsAs1DForOutWhenUnconnected=off
  wires:
  Mux1/1 -> Fcn1/1
  X/1 -> Add/1, Mux1/1
  str./1 -> Add/2, Mux1/2
  Add/1 -> Manual Switch/1
  Fcn1/1 -> Manual Switch/2
  Manual Switch/1 -> Xf/1

== system TTS2_EXT/TTS2/Pump+pipe+control valve/f2 fault ==
  X : Inport
  str. : Inport  Port=2
  Add : Sum
  Fcn : Fcn  Expr=u(1)*((u(2)/100)+1)
  Manual Switch : ManualSwitch  CurrentSetting=0
  Mux : Mux  Inputs=2
  Xf : Outport  VectorParamsAs1DForOutWhenUnconnected=off
  wires:
  Mux/1 -> Fcn/1
  X/1 -> Add/1, Mux/1
  str./1 -> Add/2, Mux/2
  Add/1 -> Manual Switch/1
  Fcn/1 -> Manual Switch/2
  Manual Switch/1 -> Xf/1

== system TTS2_EXT/TTS2/Tanks/Pipe 1-2 ==
  h1 : Inport
  k : Inport  Port=2
  h2 : Inport  Port=3
  Fcn : Fcn  Expr=sqrt(abs(u(1)*2*9.81))
  Product : Product  Inputs=3
  Sign : Signum
  Subtract : Sum  Inputs=+-
  F : Outport  VectorParamsAs1DForOutWhenUnconnected=off
  wires:
  h1/1 -> Subtract/1
  h2/1 -> Subtract/2
  Subtract/1 -> Sign/1, Fcn/1
  Fcn/1 -> Product/1
  Sign/1 -> Product/2
  k/1 -> Product/3
  Product/1 -> F/1

== system TTS2_EXT/TTS2/Tanks/Pipe 2-3 ==
  h1 : Inport
  k : Inport  Port=2
  h2 : Inport  Port=3
  Fcn : Fcn  Expr=sqrt(abs(u(1)*2*9.81))
  Product : Product  Inputs=3
  Sign : Signum
  Subtract : Sum  Inputs=+-
  F : Outport  VectorParamsAs1DForOutWhenUnconnected=off
  wires:
  h1/1 -> Subtract/1
  h2/1 -> Subtract/2
  Subtract/1 -> Sign/1, Fcn/1
  Fcn/1 -> Product/1
  Sign/1 -> Product/2
  k/1 -> Product/3
  Product/1 -> F/1

== system TTS2_EXT/TTS2/Tanks/Pipe 3-0 ==
  h1 : Inport
  k : Inport  Port=2
  h2 : Inport  Port=3
  Fcn : Fcn  Expr=sqrt(abs(u(1)*2*9.81))
  Product : Product  Inputs=3
  Sign : Signum
  Subtract : Sum  Inputs=+-
  F : Outport  VectorParamsAs1DForOutWhenUnconnected=off
  wires:
  h1/1 -> Subtract/1
  h2/1 -> Subtract/2
  Subtract/1 -> Sign/1, Fcn/1
  Fcn/1 -> Product/1
  Sign/1 -> Product/2
  k/1 -> Product/3
  Product/1 -> F/1

== system TTS2_EXT/TTS2/Tanks/Tank 1  ==
  F in : Inport
  F1 : Inport  Port=2
  A : Inport  Port=3
  kw : Inport  Port=4
  F2 : Inport  Port=5
  Divide : Product  Inputs=*/
  Gain : Gain  Gain=19.62
  Integrator : Integrator  LimitOutput=on  UpperSaturationLimit=1  LowerSaturationLimit=0
  Sqrt : Sqrt
  Subtract : Sum  Inputs=+++-
  multiply : Product  Inputs=**
  L : Outport  VectorParamsAs1DForOutWhenUnconnected=off
  wires:
  F in/1 -> Subtract/1
  F1/1 -> Subtract/2
  F2/1 -> Subtract/3
  Subtract/1 -> Divide/1
  A/1 -> Divide/2
  Divide/1 -> Integrator/1
  Integrator/1 -> Gain/1, L/1
  kw/1 -> multiply/1
  Sqrt/1 -> multiply/2
  Gain/1 -> Sqrt/1
  multiply/1 -> Subtract/4

== system TTS2_EXT/TTS2/Tanks/Tank 2 ==
  F in : Inport
  F1 : Inport  Port=2
  A : Inport  Port=3
  kw : Inport  Port=4
  F2 : Inport  Port=5
  Divide : Product  Inputs=*/
  Gain : Gain  Gain=19.62
  Integrator : Integrator  LimitOutput=on  UpperSaturationLimit=1  LowerSaturationLimit=0
  Sqrt : Sqrt
  Subtract : Sum  Inputs=+++-
  multiply : Product  Inputs=**
  L : Outport  VectorParamsAs1DForOutWhenUnconnected=off
  wires:
  F in/1 -> Subtract/1
  F1/1 -> Subtract/2
  F2/1 -> Subtract/3
  Subtract/1 -> Divide/1
  A/1 -> Divide/2
  Divide/1 -> Integrator/1
  Integrator/1 -> Gain/1, L/1
  kw/1 -> multiply/1
  Sqrt/1 -> multiply/2
  Gain/1 -> Sqrt/1
  multiply/1 -> Subtract/4

== system TTS2_EXT/TTS2/Tanks/Tank 3 ==
  F in : Inport
  F1 : Inport  Port=2
  A : Inport  Port=3
  kw : Inport  Port=4
  F2 : Inport  Port=5
  Divide : Product  Inputs=*/
  Gain : Gain  Gain=19.62
  Integrator : Integrator  LimitOutput=on  UpperSaturationLimit=1  LowerSaturationLimit=0
  Sqrt : Sqrt
  Subtract : Sum  Inputs=+++-
  multiply : Product  Inputs=**
  L : Outport  VectorParamsAs1DForOutWhenUnconnected=off
  wires:
  F in/1 -> Subtract/1
  F1/1 -> Subtract/2
  F2/1 -> Subtract/3
  Subtract/1 -> Divide/1
  A/1 -> Divide/2
  Divide/1 -> Integrator/1
  Integrator/1 -> Gain/1, L/1
  kw/1 -> multiply/1
  Sqrt/1 -> multiply/2
  Gain/1 -> Sqrt/1
  multiply/1 -> Subtract/4

== system TTS2_EXT/TTS2/Tanks/f55 fault ==
  X : Inport
  str. : Inport  Port=2
  Logical Operator : Logic  Operator=NOT  AllPortsSameDT=off  OutDataTypeStr=boolean
  Switch2 : Switch  Criteria=u2 > Threshold  SaturateOnIntegerOverflow=off  InputSameDT=off
  X' : Outport  VectorParamsAs1DForOutWhenUnconnected=off
  wires:
  Switch2/1 -> X'/1
  str./1 -> Switch2/2
  X/1 -> Switch2/3, Logical Operator/1
  Logical Operator/1 -> Switch2/1

== system TTS2_EXT/Monitoring & Analysis/r4/Function Fitting Neural Network/Layer 1 ==
  "p{1}" : Inport  PortDimensions=1
      mask Display: e = 0.06;c1 = [120 230 180]/255;c2 = ([120 230 180]+0)/(256+128);c3 = ([120 230 180]+128)/(256+128);patch([0 1 1 0],[0 0 1 1],c1);patch([0 1 1 1-e 1-e 0+e],[0 0 1 1-e 0+e 0+e],c2);patch([0 0 1 1-e 0+e 0+e],[0 1 1 1-e 1-e 0+e],c3);plot([0 1 1 0 0],[0 0 1 1 0]);
  Delays 1 : Subsystem
      mask Display: e = 0.06;c1 = [120 150 230]/255;c2 = ([120 150 230]+0)/383;c3 = ([120 150 230]+128)/383;patch([0 1 1 0],[0 0 1 1],c1);patch([0 1 1 1-e 1-e 0+e],[0 0 1 1-e 0+e 0+e],c2);patch([0 0 1 1-e 0+e 0+e],[0 1 1 1-e 1-e 0+e],c3);plot([0 1 1 0 0],[0 0 1 1 0]);disp('0');
  "IW{1,1}" : Subsystem
      mask Display: e = 0.06;c1 = [120 150 230]/255;c2 = ([120 150 230]+0)/383;c3 = ([120 150 230]+128)/383;patch([0 1 1 0],[0 0 1 1],c1);patch([0 1 1 1-e 1-e 0+e],[0 0 1 1-e 0+e 0+e],c2);patch([0 0 1 1-e 0+e 0+e],[0 1 1 1-e 1-e 0+e],c3);plot([0 1 1 0 0],[0 0 1 1 0]);disp('W');
  "b{1}" : Constant  Value=[12.5595032628997866908093783422373235225677490234375;9.0137408913545211675000246032141149044036865234375;-5.99437740726605117203007466741837561130523681640625;-4.31427156863327265767793505801819264888763427734375;0.23078101359262970238006573708844371140003204345703125;-1.3307554044509910529114904420566745102405548095703125;-3.269583881676725756193491179146803915500640869140625;-4.22281736818375730280195057275705039501190185546875;-10.9485419073701226722050705575384199619293212890625;17.15112561779046274068605271168053150177001953125]
      mask Display: e = 0.06;c1 = [120 150 230]/255;c2 = ([120 150 230]+0)/383;c3 = ([120 150 230]+128)/383;patch([0 1 1 0],[0 0 1 1],c1);patch([0 1 1 1-e 1-e 0+e],[0 0 1 1-e 0+e 0+e],c2);patch([0 0 1 1-e 0+e 0+e],[0 1 1 1-e 1-e 0+e],c3);plot([0 1 1 0 0],[0 0 1 1 0]);disp('b');
  netsum : Sum  Inputs=2  InputSameDT=on  SaturateOnIntegerOverflow=on  OutDataTypeStr=Inherit: Same as first input
      mask Display: e = 0.06;c1 = [120 150 230]/255;c2 = ([120 150 230]+0)/383;c3 = ([120 150 230]+128)/383;patch([0 1 1 0],[0 0 1 1],c1);patch([0 1 1 1-e 1-e 0+e],[0 0 1 1-e 0+e 0+e],c2);patch([0 0 1 1-e 0+e 0+e],[0 1 1 1-e 1-e 0+e],c3);plot([0 1 1 0 0],[0 0 1 1 0]);disp('+');
  tansig : neural/Transfer Functions/tansig
  "a{1}" : Outport  InitialOutput=[0;0;0;0;0;0;0;0;0;0]
      mask Display: e = 0.06;c1 = [120 230 180]/255;c2 = ([120 230 180]+0)/(256+128);c3 = ([120 230 180]+128)/(256+128);patch([0 1 1 0],[0 0 1 1],c1);patch([0 1 1 1-e 1-e 0+e],[0 0 1 1-e 0+e 0+e],c2);patch([0 0 1 1-e 0+e 0+e],[0 1 1 1-e 1-e 0+e],c3);plot([0 1 1 0 0],[0 0 1 1 0]);
  wires:
  "p{1}"/1 -> Delays 1/1("p{1}")
  Delays 1/1("pd{1,1}") -> "IW{1,1}"/1("pd{1,1}")
  "IW{1,1}"/1("iz{1,1}") -> netsum/1
  "b{1}"/1 -> netsum/2
  netsum/1 -> tansig/1
  tansig/1 -> "a{1}"/1

== system TTS2_EXT/Monitoring & Analysis/r4/Function Fitting Neural Network/Layer 2 ==
  "a{1} " : Inport  PortDimensions=10
      mask Display: e = 0.06;c1 = [120 230 180]/255;c2 = ([120 230 180]+0)/(256+128);c3 = ([120 230 180]+128)/(256+128);patch([0 1 1 0],[0 0 1 1],c1);patch([0 1 1 1-e 1-e 0+e],[0 0 1 1-e 0+e 0+e],c2);patch([0 0 1 1-e 0+e 0+e],[0 1 1 1-e 1-e 0+e],c3);plot([0 1 1 0 0],[0 0 1 1 0]);
  Delays 1 : Subsystem
      mask Display: e = 0.06;c1 = [120 150 230]/255;c2 = ([120 150 230]+0)/383;c3 = ([120 150 230]+128)/383;patch([0 1 1 0],[0 0 1 1],c1);patch([0 1 1 1-e 1-e 0+e],[0 0 1 1-e 0+e 0+e],c2);patch([0 0 1 1-e 0+e 0+e],[0 1 1 1-e 1-e 0+e],c3);plot([0 1 1 0 0],[0 0 1 1 0]);disp('0');
  "LW{2,1}" : Subsystem
      mask Display: e = 0.06;c1 = [120 150 230]/255;c2 = ([120 150 230]+0)/383;c3 = ([120 150 230]+128)/383;patch([0 1 1 0],[0 0 1 1],c1);patch([0 1 1 1-e 1-e 0+e],[0 0 1 1-e 0+e 0+e],c2);patch([0 0 1 1-e 0+e 0+e],[0 1 1 1-e 1-e 0+e],c3);plot([0 1 1 0 0],[0 0 1 1 0]);disp('W');
  "b{2}" : Constant  Value=-1.476985233725619739431067500845529139041900634765625
      mask Display: e = 0.06;c1 = [120 150 230]/255;c2 = ([120 150 230]+0)/383;c3 = ([120 150 230]+128)/383;patch([0 1 1 0],[0 0 1 1],c1);patch([0 1 1 1-e 1-e 0+e],[0 0 1 1-e 0+e 0+e],c2);patch([0 0 1 1-e 0+e 0+e],[0 1 1 1-e 1-e 0+e],c3);plot([0 1 1 0 0],[0 0 1 1 0]);disp('b');
  netsum : Sum  Inputs=2  InputSameDT=on  SaturateOnIntegerOverflow=on  OutDataTypeStr=Inherit: Same as first input
      mask Display: e = 0.06;c1 = [120 150 230]/255;c2 = ([120 150 230]+0)/383;c3 = ([120 150 230]+128)/383;patch([0 1 1 0],[0 0 1 1],c1);patch([0 1 1 1-e 1-e 0+e],[0 0 1 1-e 0+e 0+e],c2);patch([0 0 1 1-e 0+e 0+e],[0 1 1 1-e 1-e 0+e],c3);plot([0 1 1 0 0],[0 0 1 1 0]);disp('+');
  purelin : neural/Transfer Functions/purelin
  "a{2}" : Outport  InitialOutput=0
      mask Display: e = 0.06;c1 = [120 230 180]/255;c2 = ([120 230 180]+0)/(256+128);c3 = ([120 230 180]+128)/(256+128);patch([0 1 1 0],[0 0 1 1],c1);patch([0 1 1 1-e 1-e 0+e],[0 0 1 1-e 0+e 0+e],c2);patch([0 0 1 1-e 0+e 0+e],[0 1 1 1-e 1-e 0+e],c3);plot([0 1 1 0 0],[0 0 1 1 0]);
  wires:
  "a{1} "/1 -> Delays 1/1("p{2}")
  Delays 1/1("pd{2,1}") -> "LW{2,1}"/1("ad{2,1}")
  "LW{2,1}"/1("lz{2,1}") -> netsum/1
  "b{2}"/1 -> netsum/2
  netsum/1 -> purelin/1
  purelin/1 -> "a{2}"/1

== system TTS2_EXT/Monitoring & Analysis/r4/Function Fitting Neural Network/Process Input 1 ==
  x : Inport  PortDimensions=1
      mask Display: e = 0.06;c1 = [120 230 180]/255;c2 = ([120 230 180]+0)/(256+128);c3 = ([120 230 180]+128)/(256+128);patch([0 1 1 0],[0 0 1 1],c1);patch([0 1 1 1-e 1-e 0+e],[0 0 1 1-e 0+e 0+e],c2);patch([0 0 1 1-e 0+e 0+e],[0 1 1 1-e 1-e 0+e],c3);plot([0 1 1 0 0],[0 0 1 1 0]);
  mapminmax : neural/Processing Functions/mapminmax  xmin=-0.000236846370144925318784734358246  xmax=0.396988688383906829226788204323  ymin=-1  ymax=1
  p : Outport  PortDimensions=1
      mask Display: e = 0.06;c1 = [120 230 180]/255;c2 = ([120 230 180]+0)/(256+128);c3 = ([120 230 180]+128)/(256+128);patch([0 1 1 0],[0 0 1 1],c1);patch([0 1 1 1-e 1-e 0+e],[0 0 1 1-e 0+e 0+e],c2);patch([0 0 1 1-e 0+e 0+e],[0 1 1 1-e 1-e 0+e],c3);plot([0 1 1 0 0],[0 0 1 1 0]);
  wires:
  x/1 -> mapminmax/1
  mapminmax/1 -> p/1

== system TTS2_EXT/Monitoring & Analysis/r4/Function Fitting Neural Network/Process Output 1 ==
  a : Inport  PortDimensions=1
      mask Display: e = 0.06;c1 = [120 230 180]/255;c2 = ([120 230 180]+0)/(256+128);c3 = ([120 230 180]+128)/(256+128);patch([0 1 1 0],[0 0 1 1],c1);patch([0 1 1 1-e 1-e 0+e],[0 0 1 1-e 0+e 0+e],c2);patch([0 0 1 1-e 0+e 0+e],[0 1 1 1-e 1-e 0+e],c3);plot([0 1 1 0 0],[0 0 1 1 0]);
  mapminmax_reverse : neural/Processing Functions/mapminmax_reverse  xmin=-0.193966527130200377948554546492  xmax=27.2201044919786632192426623078  ymin=-1  ymax=1
  y : Outport  PortDimensions=1
      mask Display: e = 0.06;c1 = [120 230 180]/255;c2 = ([120 230 180]+0)/(256+128);c3 = ([120 230 180]+128)/(256+128);patch([0 1 1 0],[0 0 1 1],c1);patch([0 1 1 1-e 1-e 0+e],[0 0 1 1-e 0+e 0+e],c2);patch([0 0 1 1-e 0+e 0+e],[0 1 1 1-e 1-e 0+e],c3);plot([0 1 1 0 0],[0 0 1 1 0]);
  wires:
  a/1 -> mapminmax_reverse/1
  mapminmax_reverse/1 -> y/1

== system TTS2_EXT/TTS2/Disturbance: Pump+pipe+control valve/VB/Positioner ==
  CV[0-100] : Inport
  Gain : Gain  Gain=0.01
  inertia : TransferFcn  Denominator=[0.1 1]
  X[0-1] : Outport  VectorParamsAs1DForOutWhenUnconnected=off
  wires:
  CV[0-100]/1 -> Gain/1
  Gain/1 -> inertia/1
  inertia/1 -> X[0-1]/1

== system TTS2_EXT/TTS2/Disturbance: Pump+pipe+control valve/VB/Valve ==
  G[0-1] : Inport
  P1[kPa] : Inport  Port=2
  P2[kPa] : Inport  Port=3
  Abs : Abs  SaturateOnIntegerOverflow=off
  Bus Creator : BusCreator  Inputs=4
  Product : Product
  Saturation : Saturate  UpperLimit=1  LowerLimit=0
  Sign : Signum
  Sum : Sum  Inputs=|+-
  Sum1 : Sum  Inputs=|+-
  Switch : Switch  Criteria=u2 > Threshold  SaturateOnIntegerOverflow=off  InputSameDT=off
  Transfer Fcn : TransferFcn  Denominator=[1 1]
  alfa : Constant
  kv_max : Constant  Value=0.000075
  lin_range : Constant
  liniowa : Subsystem
  ro : Constant
  stałoproc. : Subsystem
  F[m3/h] : Outport  VectorParamsAs1DForOutWhenUnconnected=off
  wires:
  G[0-1]/1 -> Saturation/1
  Saturation/1 -> liniowa/1(CV), stałoproc./1(CV), Sum/1
  P1[kPa]/1 -> Sum1/1
  P2[kPa]/1 -> Sum1/2
  Sum1/1 -> Sign/1, Abs/1
  kv_max/1 -> Bus Creator/1
  alfa/1 -> Bus Creator/2
  lin_range/1 -> Bus Creator/4, Sum/2
  ro/1 -> Bus Creator/3
  Switch/1 -> Product/1
  Product/1 -> Transfer Fcn/1
  Transfer Fcn/1 -> F[m3/h]/1
  Bus Creator/1 -> liniowa/3(param), stałoproc./3(param)
  Abs/1 -> liniowa/2(dP), stałoproc./2(dP)
  Sum/1 -> Switch/2
  Sign/1 -> Product/2
  stałoproc./1(F) -> Switch/1
  liniowa/1(F) -> Switch/3

== system TTS2_EXT/TTS2/Pump+pipe+control valve/V1/Positioner ==
  CV[0-100] : Inport
  Gain : Gain  Gain=0.01
  Saturation : Saturate  UpperLimit=1  LowerLimit=0
  inertia : TransferFcn  Denominator=[0.1 1]
  X[0-1] : Outport  VectorParamsAs1DForOutWhenUnconnected=off
  wires:
  CV[0-100]/1 -> Gain/1
  Gain/1 -> inertia/1
  inertia/1 -> Saturation/1
  Saturation/1 -> X[0-1]/1

== system TTS2_EXT/TTS2/Pump+pipe+control valve/V1/Valve ==
  G[0-1] : Inport
  P1[kPa] : Inport  Port=2
  P2[kPa] : Inport  Port=3
  Abs : Abs  SaturateOnIntegerOverflow=off
  Bus Creator : BusCreator  Inputs=4
  Product : Product
  Saturation : Saturate  UpperLimit=1  LowerLimit=0
  Sign : Signum
  Sum : Sum  Inputs=|+-
  Sum1 : Sum  Inputs=|+-
  Switch : Switch  Criteria=u2 > Threshold  SaturateOnIntegerOverflow=off  InputSameDT=off
  Transfer Fcn : TransferFcn  Denominator=[1 1]
  alfa : Constant  Value=2
  kv_max : Constant  Value=0.00049
  lin_range : Constant  Value=0.1
  liniowa : Subsystem
  ro : Constant
  stałoproc. : Subsystem
  dP[kPa] : Outport  VectorParamsAs1DForOutWhenUnconnected=off
  F[m3/s] : Outport  Port=2  VectorParamsAs1DForOutWhenUnconnected=off
  wires:
  G[0-1]/1 -> Saturation/1
  Saturation/1 -> liniowa/1(CV), stałoproc./1(CV), Sum/1
  P1[kPa]/1 -> Sum1/1
  P2[kPa]/1 -> Sum1/2
  Sum1/1 -> dP[kPa]/1, Sign/1, Abs/1
  kv_max/1 -> Bus Creator/1
  alfa/1 -> Bus Creator/2
  lin_range/1 -> Bus Creator/4, Sum/2
  ro/1 -> Bus Creator/3
  Switch/1 -> Product/1
  Product/1 -> Transfer Fcn/1
  Transfer Fcn/1 -> F[m3/s]/1
  Bus Creator/1 -> liniowa/3(param), stałoproc./3(param)
  Abs/1 -> liniowa/2(dP), stałoproc./2(dP)
  Sum/1 -> Switch/2
  Sign/1 -> Product/2
  stałoproc./1(F) -> Switch/1
  liniowa/1(F) -> Switch/3

== system TTS2_EXT/TTS2/Pump+pipe+control valve/V1/f4 fault ==
  X : Inport
  str. : Inport  Port=2
  Add : Sum
  Fcn : Fcn  Expr=u(1)*((u(2)/100)+1)
  Manual Switch : ManualSwitch  CurrentSetting=0
  Mux : Mux  Inputs=2
  Xf : Outport  VectorParamsAs1DForOutWhenUnconnected=off
  wires:
  Mux/1 -> Fcn/1
  X/1 -> Add/1, Mux/1
  str./1 -> Add/2, Mux/2
  Add/1 -> Manual Switch/1
  Fcn/1 -> Manual Switch/2
  Manual Switch/1 -> Xf/1

== system TTS2_EXT/TTS2/Pump+pipe+control valve/V1/f6 fault ==
  X : Inport
  str. : Inport  Port=2
  Add : Sum
  Fcn : Fcn  Expr=u(1)*((u(2)/100)+1)
  Manual Switch : ManualSwitch  CurrentSetting=0
  Mux : Mux  Inputs=2
  Xf : Outport  VectorParamsAs1DForOutWhenUnconnected=off
  wires:
  Mux/1 -> Fcn/1
  X/1 -> Add/1, Mux/1
  str./1 -> Add/2, Mux/2
  Add/1 -> Manual Switch/1
  Fcn/1 -> Manual Switch/2
  Manual Switch/1 -> Xf/1

== system TTS2_EXT/TTS2/Pump+pipe+control valve/V2/Positioner ==
  CV[0-100] : Inport
  Gain : Gain  Gain=0.01
  Saturation : Saturate  UpperLimit=1  LowerLimit=0
  inertia : TransferFcn  Denominator=[0.1 1]
  X[0-1] : Outport  VectorParamsAs1DForOutWhenUnconnected=off
  wires:
  CV[0-100]/1 -> Gain/1
  Gain/1 -> inertia/1
  inertia/1 -> Saturation/1
  Saturation/1 -> X[0-1]/1

== system TTS2_EXT/TTS2/Pump+pipe+control valve/V2/Valve ==
  G[0-1] : Inport
  P1[kPa] : Inport  Port=2
  P2[kPa] : Inport  Port=3
  Abs : Abs  SaturateOnIntegerOverflow=off
  Bus Creator : BusCreator  Inputs=4
  Product : Product
  Saturation : Saturate  UpperLimit=1  LowerLimit=0
  Sign : Signum
  Sum : Sum  Inputs=|+-
  Sum1 : Sum  Inputs=|+-
  Switch : Switch  Criteria=u2 > Threshold  SaturateOnIntegerOverflow=off  InputSameDT=off
  Transfer Fcn : TransferFcn  Denominator=[1 1]
  alfa : Constant  Value=2
  kv_max : Constant  Value=0.00049
  lin_range : Constant  Value=0.1
  liniowa : Subsystem
  ro : Constant
  stałoproc. : Subsystem
  dP[kPa] : Outport  VectorParamsAs1DForOutWhenUnconnected=off
  F[m3/s] : Outport  Port=2  VectorParamsAs1DForOutWhenUnconnected=off
  wires:
  G[0-1]/1 -> Saturation/1
  Saturation/1 -> liniowa/1(CV), stałoproc./1(CV), Sum/1
  P1[kPa]/1 -> Sum1/1
  P2[kPa]/1 -> Sum1/2
  Sum1/1 -> dP[kPa]/1, Sign/1, Abs/1
  kv_max/1 -> Bus Creator/1
  alfa/1 -> Bus Creator/2
  lin_range/1 -> Bus Creator/4, Sum/2
  ro/1 -> Bus Creator/3
  Switch/1 -> Product/1
  Product/1 -> Transfer Fcn/1
  Transfer Fcn/1 -> F[m3/s]/1
  Bus Creator/1 -> liniowa/3(param), stałoproc./3(param)
  Abs/1 -> liniowa/2(dP), stałoproc./2(dP)
  Sum/1 -> Switch/2
  Sign/1 -> Product/2
  stałoproc./1(F) -> Switch/1
  liniowa/1(F) -> Switch/3

== system TTS2_EXT/TTS2/Pump+pipe+control valve/V2/f53 fault ==
  X : Inport
  str. : Inport  Port=2
  Add : Sum
  Fcn : Fcn  Expr=u(1)*((u(2)/100)+1)
  Manual Switch : ManualSwitch
  Mux : Mux  Inputs=2
  Xf : Outport  VectorParamsAs1DForOutWhenUnconnected=off
  wires:
  Mux/1 -> Fcn/1
  X/1 -> Add/1, Mux/1
  str./1 -> Add/2, Mux/2
  Add/1 -> Manual Switch/1
  Fcn/1 -> Manual Switch/2
  Manual Switch/1 -> Xf/1

== system TTS2_EXT/Monitoring & Analysis/r4/Function Fitting Neural Network/Layer 1/Delays 1 ==
  "p{1}" : Inport  PortDimensions=1
      mask Display: e = 0.06;c1 = [120 230 180]/255;c2 = ([120 230 180]+0)/(256+128);c3 = ([120 230 180]+128)/(256+128);patch([0 1 1 0],[0 0 1 1],c1);patch([0 1 1 1-e 1-e 0+e],[0 0 1 1-e 0+e 0+e],c2);patch([0 0 1 1-e 0+e 0+e],[0 1 1 1-e 1-e 0+e],c3);plot([0 1 1 0 0],[0 0 1 1 0]);
  mux : Mux  Inputs=1
      mask Display: e = 0.06;c1 = [120 150 230]/255;c2 = ([120 150 230]+0)/383;c3 = ([120 150 230]+128)/383;patch([0 1 1 0],[0 0 1 1],c1);patch([0 1 1 1-e 1-e 0+e],[0 0 1 1-e 0+e 0+e],c2);patch([0 0 1 1-e 0+e 0+e],[0 1 1 1-e 1-e 0+e],c3);plot([0 1 1 0 0],[0 0 1 1 0]);disp('Mux')
  "pd{1,1}" : Outport
      mask Display: e = 0.06;c1 = [120 230 180]/255;c2 = ([120 230 180]+0)/(256+128);c3 = ([120 230 180]+128)/(256+128);patch([0 1 1 0],[0 0 1 1],c1);patch([0 1 1 1-e 1-e 0+e],[0 0 1 1-e 0+e 0+e],c2);patch([0 0 1 1-e 0+e 0+e],[0 1 1 1-e 1-e 0+e],c3);plot([0 1 1 0 0],[0 0 1 1 0]);
  wires:
  "p{1}"/1 -> mux/1
  mux/1 -> "pd{1,1}"/1
